simulink model "Filter_Simulation1"  (R2015b)
settings: Solver=FixedStepDiscrete  StartTime=0.0  StopTime=4  FixedStep=0.01  RelTol=1e-3
undefined symbols (not defined in the file): dfilt, fdesignblkfcn, gcbh
libraries: dsparch4 x1, dspsrcs4 x1
settings Model: ExtModeArmWhenConnect=off  Creator=userid  LastModifiedBy=primozc
settings SolverCC: PositivePriorityOrder=on
settings DataIOCC: SaveFormat=Array  SignalLoggingSaveFormat=ModelDataLogs
settings OptimizationCC: BooleanDataType=off  OptimizeBlockIOStorage=off  BufferReuse=off  GlobalBufferReuse=off  ExpressionFolding=off  ExpressionDepthLimit=2147483647  LocalBlockOutputs=off  InitFltsAndDblsToZero=on
settings DebuggingCC: SaveWithParameterizedLinksMsg=none  UnderspecifiedInitializationDetection=Classic  MergeDetectMultiDrivingBlocksExec=none  SolverPrmCheckMsg=warning  FcnCallInpInsideContextMsg=UseLocalSettings  StateNameClashWarn=warning
settings HardwareCC: ProdBitPerPointer=32  ProdLargestAtomicFloat=None  ProdIntDivRoundTo=Undefined  ProdEndianess=Unspecified  ProdWordSize=32  ProdHWDeviceType=32-bit Generic
settings RTWCC: SystemTargetFile=quarc_windows.tlc  TemplateMakefile=quarc_default_tmf  Description=QuaRC Win32 Target
settings STFCustomTargetCC: TargetPreCompLibLocation=C:\PROGRA~3\QUARC\lib\2015b\windows\release  ConcurrentExecutionCompliant=off  SystemTargetFile=quarc_windows.tlc
settings GRTTargetCC: TargetPreCompLibLocation=C:\PROGRA~3\QUARC\lib\2015b\windows\release  ParMdlRefBuildCompliant=off  CompOptLevelCompliant=off  ConcurrentExecutionCompliant=off  GeneratePreprocessorConditionals=Disable all  CombineOutputUpdateFcns=off  MatFileLogging=off  GRTInterface=on  UseToolchainInfoCompliant=off  ExtMode=on  ExtModeMexFile=quarc_comm
settings ConfigComp: CovModelRefEnable=Off

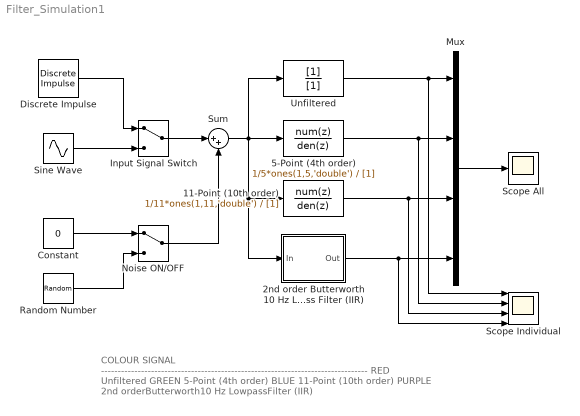
== system Filter_Simulation1 ==
  note: COLOUR SIGNAL
      | --------------------------------------------------------------------------------
      | RED Unfiltered
      | GREEN 5-Point (4th order)
      | BLUE 11-Point (10th order)
      | PURPLE 2nd orderButterworth10 Hz LowpassFilter (IIR)
  11-Point (10th order) : DiscreteFilter  Numerator=1/11*ones(1,11,'double')  Denominator=[1]
  2nd order Butterworth 10 Hz Lowpass Filter (IIR) : Subsystem  DialogController=fdesignblkfcn  InitFcn=fdesignblkfcn(gcbh, {'InitFcn'});  mask(Lowpass Filter){}
      mask help: Design a lowpass filter
      settings: CopyFcn=fdesignblkfcn(gcbh, {'CopyFcn'});
      mask Help: helpview(mapfilelocation('dsp'), 'dsplowpassfilter');
      mask Display: disp('Lowpass')
  5-Point (4th order) : DiscreteFilter  Numerator=1/5*ones(1,5,'double')  Denominator=[1]
  Constant : Constant  Value=0
  Discrete Impulse : dspsrcs4/Discrete  Impulse  Delay=100  SampleTime=0.01  FrameSample=1  OutputFrames=on  dataType=double  isSigned=on  wordLen=16  udDataType=sfix(16)  fracBitsMode=Best precision  numFracBits=15  OutDataTypeStr=double  LastOutDataTypeStr=double
  Input Signal Switch : ManualSwitch
  Mux : Mux
  Noise ON/OFF : ManualSwitch
  Random Number : RandomNumber  Variance=.2  Seed=111  SampleTime=.01
  Scope All : Scope
  Scope Individual : Scope  NumInputPorts=4
  Sine Wave : Sin  Amplitude=4  Frequency=1*2*pi  SampleTime=0.01
  Sum : Sum  Inputs=|++
  Unfiltered : DiscreteFilter  Denominator=[1]
  wires:
  Sum/1 -> 11-Point (10th order)/1, 2nd order Butterworth 10 Hz Lowpass Filter (IIR)/1(In), 5-Point (4th order)/1, Unfiltered/1
  Unfiltered/1 -> Mux/1, Scope Individual/1
  5-Point (4th order)/1 -> Mux/2, Scope Individual/2
  11-Point (10th order)/1 -> Mux/3, Scope Individual/3
  2nd order Butterworth 10 Hz Lowpass Filter (IIR)/1(Out) -> Mux/4, Scope Individual/4
  Mux/1 -> Scope All/1
  Discrete Impulse/1 -> Input Signal Switch/1
  Sine Wave/1 -> Input Signal Switch/2
  Input Signal Switch/1 -> Sum/1
  Constant/1 -> Noise ON/OFF/1
  Random Number/1 -> Noise ON/OFF/2
  Noise ON/OFF/1 -> Sum/2

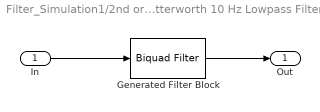
== system Filter_Simulation1/2nd order Butterworth 10 Hz Lowpass Filter (IIR) ==
  In : Inport
  Generated Filter Block : dsparch4/Biquad Filter  Tag=BlockMethodSubSystem  IIRFiltStruct=Direct form II  CoeffSource=Specify via dialog  BiQuadCoeffs=[0.25138933796645635 0.5027786759329127 0.25138933796645635 1 -1.1429805025399009 0.41280159809618855]  a0Flag=Warning  IC=0  ICnum=0  ICden=0  InputProcessing=Columns as channels (frame based)  denAccumFracLength=30  denProdOutputFracLength=30  secondMemoryFracLength=15  roundingMode=Floor  overflowMode=off  ScaleValues=[0.26832989193070972;1]  optimizeScaleValues=off  ScaleValueMode=Specify via input port (g)  scaleValueFracLength=14  FilterSource=Specify via dialog  FilterObject=dfilt.df2tsos([1 0.3 0.4],[1 0.1 0.2])
  Out : Outport
  wires:
  In/1 -> Generated Filter Block/1
  Generated Filter Block/1 -> Out/1
